simulink model "simulation"  (R2021b)
settings: Solver=VariableStepAuto  StartTime=0.0  StopTime=10.0  MaxStep=0.001  RelTol=1e-3
settings Model: Creator=ze  LastModifiedBy=pedro

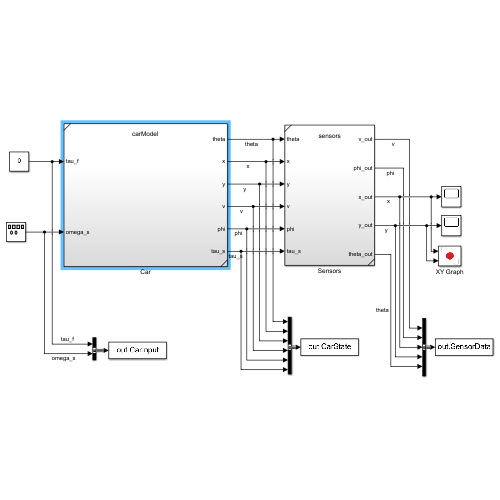
[thumbnail: Simulink's stored preview of the top-level diagram]
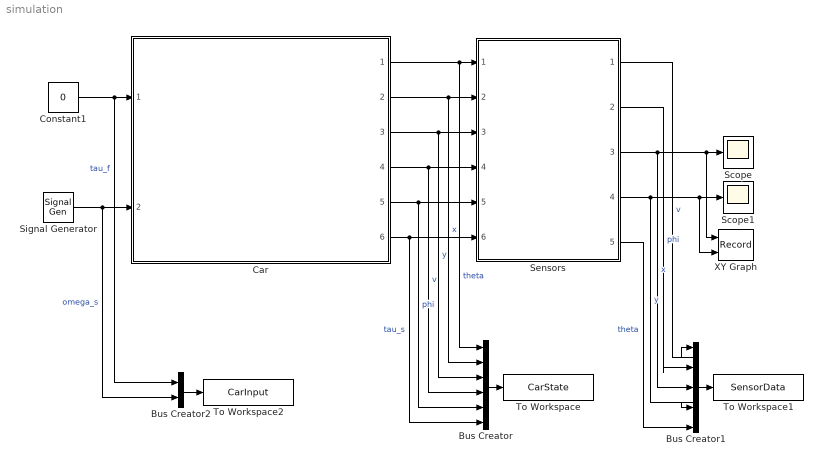
== system simulation ==
  Bus Creator : BusCreator  Inputs=6
  Bus Creator1 : BusCreator  Inputs=5
  Bus Creator2 : BusCreator  Inputs=2
  Car : Subsystem  ReferencedSubsystem=carModel
  Constant1 : Constant  Value=0
  Scope : Scope
  Scope1 : Scope
  Sensors : Subsystem  ReferencedSubsystem=sensors
  Signal Generator : SignalGenerator  Amplitude=pi/4  Frequency=0.001  Units=rad/sec
  To Workspace : ToWorkspace  VariableName=CarState  SaveFormat=Timeseries  SampleTime=-1
  To Workspace1 : ToWorkspace  VariableName=SensorData  SaveFormat=Timeseries  SampleTime=-1
  To Workspace2 : ToWorkspace  VariableName=CarInput  SaveFormat=Timeseries  SampleTime=-1
  XY Graph : Record  FileSettingsInternal="{\"entries\":[{\"content\":{\"excelSettings\":{\"content\":{},\"type\":\"Streamout.ExcelSettings\"}},\"type\":\"Streamout.FileSettingStorage\",\"uuid\":\"50900d95-aa02-4ba2-a71a-ae1540d2eb9a\"}],\"packageUris\":[\"http://schema.mathworks.com/mf0/streamout_blocks/R2020a\"],\"version\":\"1.0\"}"  Layout=[1 1]  SignalsInternal="{\"entries\":[{\"content\":{\"signals\":[{\"content\":{\"blockPath\":[\"simulation/XY Graph\"],\"channel\":[],\"dimensions\":[1],\"domain\":\"simulation/XY Graph\",\"lineColor\":\"#a2142f\",\"plots\":[1],\"port\":1,\"sid\":[\"\"],\"signalID\":22,\"signalName\":\"Sensors:3\"},\"type\":\"RecordBlkView.Signal\",\"uuid\":\"8a27b2f1-bc9f-40b2-9969-70aa7b5809b1\"},{\"content\":{\"blockPath\":[\"simulation/XY Graph\"],\"channel\":[],\"dimensions\":[1],\"domain\":\"simulation/XY Graph\",\"lineColor\":\"#139fff\",\"plots\":[1],\"port\":2,\"sid\":[\"\"],\"signalID\":26,\"signalName\":\"Sensors:4\"},\"type\":\"RecordBlkView.Signal\",\"uuid\":\"c422a81e-d649-4a6e-8105-2367932bcd93\"}]},\"type\":\"RecordBlkView.InputSignals\",\"uuid\":\"ee2b27a4-ab58-40e7-be5b-b2f191ccf998\"}],\"packageUris\":[\"http://schema.mathworks.com/mf0/streamout_blocks/R2020a\"],\"version\":\"1.0\"}"  VisualizationBindings="{\"xyplotplugin\":{\"info\":[{\"series\":[{\"bindingParametersList\":[{\"parameter\":\"X-Axis\",\"signalID\":22,\"signalName\":\"Sensors:3\"},{\"parameter\":\"Y-Axis\",\"signalID\":26,\"signalName\":\"Sensors:4\"}],\"seriesID\":40482}],\"subplotID\":1}]}}"  CompatibilityTag=XY
  wires:
  Car/1 -> Bus Creator/1, Sensors/1  "theta"
  Car/2 -> Bus Creator/2, Sensors/2  "x"
  Car/3 -> Bus Creator/3, Sensors/3  "y"
  Car/4 -> Bus Creator/4, Sensors/4  "v"
  Car/5 -> Bus Creator/5, Sensors/5  "phi"
  Car/6 -> Bus Creator/6, Sensors/6  "tau_s"
  Sensors/3 -> Bus Creator1/3, XY Graph/1, Scope/1  "x"
  Constant1/1 -> Bus Creator2/1, Car/1  "tau_f"
  Signal Generator/1 -> Bus Creator2/2, Car/2  "omega_s"
  Sensors/4 -> Bus Creator1/4, XY Graph/2, Scope1/1  "y"
  Bus Creator/1 -> To Workspace/1
  Sensors/1 -> Bus Creator1/1  "v"
  Sensors/2 -> Bus Creator1/2  "phi"
  Sensors/5 -> Bus Creator1/5  "theta"
  Bus Creator1/1 -> To Workspace1/1
  Bus Creator2/1 -> To Workspace2/1
